simulink model "VCU_SW"  (R2020b)
settings: Solver=FixedStepDiscrete  StartTime=0.0  StopTime=inf  FixedStep=1e-2  RelTol=1e-3
PreLoadFcn:
  | RTWConfigurationCB('preloadfcn', bdroot);
InitFcn:
  | loadvar_ttc500
undefined symbols (not defined in the file): BrkPedalTypes, CabMovModeTypes, cFuseTempSensAcc_X, cFuseTempSensAcc_Y, cFuseTempSensVal_X, cFuseTempSensVal_Y, cTMSTempSensVal_X, cTMSTempSensVal_Y, cTransferCaseSpeedRatio, diag_state, DoorsPositionTypes, dP_filter_Y, DriverOccClassSystemTypes, ErrorValueTypes, fatal_error_callback, IO_ADC_NO_RANGE, LadderStatusTypes, pAnalogCabRotSensAcc, pAnalogCabRotSensMaxVolt, pAnalogCabRotSensMinVolt, pAnalogCabRotSensRange, pAnalogCabRotSensZeroVolt, pBrkActivePress, pCabTiltSensAcc, pCabTiltSensMaxCur, pCabTiltSensMinCur, pDistanceCorrection, pECANManual_BPNEnable, pECANManual_BPNEnabler_Flag, pFilterSensAccRes, pHDirMaxDiffFrq, pHDirSensHighLvl, pHDirSensLowLvl, pMainGearRatio, pMaxFilterSensRes, pMaxFirstPedalSensValue, pMaxFuseTempSensRes, pMaxPressLoss, pMaxPressSensCurrent, pMaxPressValue, pMaxPressValueHydMotAndPump, pMaxPressValueParkDrain, pMaxSecondPedalSensValue, pMaxTempSensVoltage, pMaxTempValue, pMaxTMSTempSensRes, pMinFilterSensRes, pMinFirstPedalSensValue, pMinFuseTempSensRes, pMinPressLoss, pMinPressSensCurrent, pMinPressValue, pMinSecondPedalSensValue, pMinTempSensVoltage, pMinTempValue, pMinTMSTempSensRes, pMotorRingTeethNum, pPedalSensAccuracyPct, pPedalSensAccuracyVolt, pPressLossTreshhold ... (+20)
libraries: TTlibrary x270, canmsglib x127, simulink x88
(part 11 of 17)

== system VCU_SW/InputLayer/InputNetwork/InputCCAN/GetCCAN100msec/CM3 ==
  CAN_Unpack_Cab_CM3 : canmsglib/CAN Unpack  MsgList=(none)  MsgName=CM3  MsgIDType=Extended (29-bit identifier)  MsgIdentifier=419288069  MsgLength=8  SignalInfo={ 'Transfer_Case_Selector_Switch', '0', '3', 'LE', 'unsigned', 'Standard', '0', '1', '0', '0', '7' }  IDPort=off  TimestampPort=off  ErrorPort=off  RemotePort=off  LengthPort=off  StatusPort=off  ApplyMinMax=off
      settings: SourceProductBaseCode=ME,XP,VN
  DataStoreWrite_PLC_StateM : DataStoreWrite  DataStoreName=InputNetworkData  DataStoreElements=InputNetworkData.CCAN.CM3.Transfer_Case_Selector_Switch
  MATLAB Function : MATLAB Function  TreatAsAtomicUnit=on
  Terminator : Terminator
  read_message_Cab_CM3 : TTlibrary/CAN/read_message_name  channel=IO_CAN_CHANNEL_1  id_format=IO_CAN_EXT_FRAME  get_msg_info=off  message_names=there is no CAN Unpack blocks  message_info=|  id=419288069  ac_mask=536870911  retranslation=off  io_error=on  sample_time=-1
      | Message Name: CM3
      |  Message ID Type: Extended (29-bit identifier)
      |  Message ID: 419288069
      settings: SourceProductName=TT control 500 series
  wires:
  MATLAB Function/1(TransferCaseEnum) -> DataStoreWrite_PLC_StateM/1
  CAN_Unpack_Cab_CM3/1 -> MATLAB Function/1(value)
  read_message_Cab_CM3/1 -> CAN_Unpack_Cab_CM3/1  "msg_419288069"
  read_message_Cab_CM3/2 -> Terminator/1  "handler_err_419288069"

== system VCU_SW/InputLayer/InputNetwork/InputCCAN/GetCCAN100msec/CabinAuxiliaryStatus ==
  CAN_Unpack_CabinAuxiliaryStatus : canmsglib/CAN Unpack  MsgList=(none)  MsgName=CabinAuxiliaryStatus  MsgIDType=Extended (29-bit identifier)  MsgIdentifier=419376638  MsgLength=8  SignalInfo={ 'FrameLockSts', '2', '2', 'LE', 'unsigned', 'Standard', '0', '1', '0', '0', '3'; 'FuelTankStatus', '0', '2', 'LE', 'unsigned', 'Standard', '0', '1', '0', '0', '3'; 'LadderStatus', '4', '2', 'LE', 'unsigned', 'Standard', '0', '1', '0', '0', '3' }  IDPort=off  TimestampPort=off  ErrorPort=off  RemotePort=off  LengthPort=off  StatusPort=off  ApplyMinMax=off
      settings: SourceProductBaseCode=ME,XP,VN
  DataStoreWrite_PLC_StateM : DataStoreWrite  DataStoreName=InputNetworkData  DataStoreElements=InputNetworkData.CCAN.CabinAuxiliaryStatus.FrameLockStatus#InputNetworkData.CCAN.CabinAuxiliaryStatus.FuelTankStatus#InputNetworkData.CCAN.CabinAuxiliaryStatus.LadderStatus
  Enumerated Constant1 : simulink/Sources/Enumerated Constant  OutDataTypeStr=Enum: StateModeTypes  Value=StateModeTypes.STT_DISABLE  SampleTime=inf
  Enumerated Constant8 : simulink/Sources/Enumerated Constant  OutDataTypeStr=Enum: LadderStatusTypes  Value=LadderStatusTypes.LADDER_UP  SampleTime=inf
  Function Caller1 : FunctionCaller  FunctionPrototype=rawValue = convUintPinToenumStt(uintValue)  InputArgumentSpecifications=<Enter example>  OutputArgumentSpecifications=<Enter example>
  Function Caller3 : FunctionCaller  FunctionPrototype=rawValue = convUintPinToenumStt(uintValue)  InputArgumentSpecifications=<Enter example>  OutputArgumentSpecifications=<Enter example>
  MATLAB Function : MATLAB Function  TreatAsAtomicUnit=on
  Terminator : Terminator
  read_message_CabinAuxiliaryStatus : TTlibrary/CAN/read_message_name  channel=IO_CAN_CHANNEL_1  id_format=IO_CAN_EXT_FRAME  get_msg_info=off  message_names=there is no CAN Unpack blocks  message_info=|  id=419376638  ac_mask=536870911  retranslation=off  io_error=on  sample_time=-1
      | Message Name: InstrumentClusterStatus
      |  Message ID Type: Extended (29-bit identifier)
      |  Message ID: 419384087
      settings: SourceProductName=TT control 500 series
  wires:
  read_message_CabinAuxiliaryStatus/2 -> Terminator/1  "handler_err_419376638"
  read_message_CabinAuxiliaryStatus/1 -> CAN_Unpack_CabinAuxiliaryStatus/1  "msg_419376638"
  CAN_Unpack_CabinAuxiliaryStatus/1 -> Function Caller3/1
  CAN_Unpack_CabinAuxiliaryStatus/3 -> MATLAB Function/1(Value)
  CAN_Unpack_CabinAuxiliaryStatus/2 -> Function Caller1/1
  Enumerated Constant1/1 -> DataStoreWrite_PLC_StateM/1
  Function Caller1/1 -> DataStoreWrite_PLC_StateM/2
  Enumerated Constant8/1 -> DataStoreWrite_PLC_StateM/3

== system VCU_SW/InputLayer/InputNetwork/InputCCAN/GetCCAN100msec/DC1 ==
  CAN_Unpack_Cab_DC1 : canmsglib/CAN Unpack  MsgList=(none)  MsgName=DC1  MsgIDType=Extended (29-bit identifier)  MsgIdentifier=419319550  MsgLength=8  SignalInfo={ 'PositionOfDoors', '0', '4', 'LE', 'unsigned', 'Standard', '0', '1', '0', '0', '15' }  IDPort=off  TimestampPort=off  ErrorPort=off  RemotePort=off  LengthPort=off  StatusPort=off  ApplyMinMax=off
      settings: SourceProductBaseCode=ME,XP,VN
  Data Store Write : DataStoreWrite  DataStoreName=InputFunctionsData  DataStoreElements=InputFunctionsData.doorIsClosed
  DataStoreWrite_PLC_StateM : DataStoreWrite  DataStoreName=InputNetworkData  DataStoreElements=InputNetworkData.CCAN.DC1.PositionOfDoors
  Enumerated Constant : simulink/Sources/Enumerated Constant  OutDataTypeStr=Enum: DoorsPositionTypes  Value=DoorsPositionTypes.DOORS_POS_ALL_DOORS_CLOSED  SampleTime=inf
  Enumerated Constant1 : simulink/Sources/Enumerated Constant  OutDataTypeStr=Enum: DoorsPositionTypes  Value=DoorsPositionTypes.DOORS_POS_ALL_DOORS_CLOSED  SampleTime=inf
  Enumerated Constant2 : simulink/Sources/Enumerated Constant  OutDataTypeStr=Enum: StateModeTypes  Value=StateModeTypes.STT_DISABLE  SampleTime=inf
  Enumerated Constant3 : simulink/Sources/Enumerated Constant  OutDataTypeStr=Enum: StateModeTypes  Value=StateModeTypes.STT_ENABLE  SampleTime=inf
  MATLAB Function : MATLAB Function  TreatAsAtomicUnit=on
  Multiport Switch : MultiPortSwitch  DataPortOrder=Zero-based contiguous  Inputs=2  zeroidx=on
  Relational Operator : RelationalOperator  Operator===  OutDataTypeStr=boolean  RndMeth=Simplest
  Terminator : Terminator
  read_message_Cab_DC1 : TTlibrary/CAN/read_message_name  channel=IO_CAN_CHANNEL_1  id_format=IO_CAN_EXT_FRAME  get_msg_info=off  message_names=there is no CAN Unpack blocks  message_info=|  id=419319550  ac_mask=536870911  retranslation=off  io_error=on  sample_time=-1
      | Message Name: DC1
      |  Message ID Type: Extended (29-bit identifier)
      |  Message ID: 419319550
      settings: SourceProductName=TT control 500 series
  wires:
  CAN_Unpack_Cab_DC1/1 -> MATLAB Function/1(Value)
  read_message_Cab_DC1/1 -> CAN_Unpack_Cab_DC1/1  "msg_419319550"
  read_message_Cab_DC1/2 -> Terminator/1  "handler_err_419319550"
  Enumerated Constant2/1 -> Multiport Switch/2
  Multiport Switch/1 -> Data Store Write/1  "closedDoorSensState"
  Relational Operator/1 -> Multiport Switch/1
  Enumerated Constant/1 -> DataStoreWrite_PLC_StateM/1, Relational Operator/1
  Enumerated Constant1/1 -> Relational Operator/2
  Enumerated Constant3/1 -> Multiport Switch/3  "closedDoorSensState"

== system VCU_SW/InputLayer/InputNetwork/InputCCAN/GetCCAN100msec/Fan Rotation Direction Control  ==
  CAN_Unpack_Cab_FanRotationDirectionControl : canmsglib/CAN Unpack  MsgList=(none)  MsgName=FanRotationDirectionControl  MsgIDType=Extended (29-bit identifier)  MsgIdentifier=419375365  MsgLength=8  SignalInfo={ 'FanDirectCmd', '0', '2', 'LE', 'unsigned', 'Standard', '0', '1', '0', '0', '3'; 'FanReverseCmd', '2', '2', 'LE', 'unsigned', 'Standard', '0', '1', '0', '0', '3' }  IDPort=off  TimestampPort=off  ErrorPort=off  RemotePort=off  LengthPort=off  StatusPort=off  ApplyMinMax=off
      settings: SourceProductBaseCode=ME,XP,VN
  DataStoreWrite_PLC_StateM : DataStoreWrite  DataStoreName=InputNetworkData  DataStoreElements=InputNetworkData.CCAN.FanRotationDirectionControl.FanDirectCmd#InputNetworkData.CCAN.FanRotationDirectionControl.FanReverseCmd
  Function Caller1 : FunctionCaller  FunctionPrototype=rawValue = convUintPinToenumStt(uintValue)  InputArgumentSpecifications=<Enter example>  OutputArgumentSpecifications=<Enter example>
  Function Caller2 : FunctionCaller  FunctionPrototype=rawValue = convUintPinToenumStt(uintValue)  InputArgumentSpecifications=<Enter example>  OutputArgumentSpecifications=<Enter example>
  Terminator : Terminator
  read_message_Cab_FanRotationDirectionControl : TTlibrary/CAN/read_message_name  channel=IO_CAN_CHANNEL_1  id_format=IO_CAN_EXT_FRAME  get_msg_info=off  message_names=there is no CAN Unpack blocks  message_info=|  id=419375365  ac_mask=536870911  retranslation=off  io_error=on  sample_time=-1
      | Message Name: FanRotationDirectionControl
      |  Message ID Type: Extended (29-bit identifier)
      |  Message ID: 419375365
      settings: SourceProductName=TT control 500 series
  wires:
  Function Caller2/1 -> DataStoreWrite_PLC_StateM/2
  Function Caller1/1 -> DataStoreWrite_PLC_StateM/1
  CAN_Unpack_Cab_FanRotationDirectionControl/2 -> Function Caller2/1
  CAN_Unpack_Cab_FanRotationDirectionControl/1 -> Function Caller1/1
  read_message_Cab_FanRotationDirectionControl/1 -> CAN_Unpack_Cab_FanRotationDirectionControl/1  "msg_419375365"
  read_message_Cab_FanRotationDirectionControl/2 -> Terminator/1  "handler_err_419375365"

== system VCU_SW/InputLayer/InputNetwork/InputCCAN/GetCCAN100msec/Fan Rotation Direction Status  ==
  CAN_Unpack_Cab_FanRotationDirectionStatus : canmsglib/CAN Unpack  MsgList=(none)  MsgName=FanRotationDirectionStatus  MsgIDType=Extended (29-bit identifier)  MsgIdentifier=419377150  MsgLength=8  SignalInfo={ 'FanDirectSts', '0', '2', 'LE', 'unsigned', 'Standard', '0', '1', '0', '0', '3'; 'FanReverseSts', '2', '2', 'LE', 'unsigned', 'Standard', '0', '1', '0', '0', '3' }  IDPort=off  TimestampPort=off  ErrorPort=off  RemotePort=off  LengthPort=off  StatusPort=off  ApplyMinMax=off
      settings: SourceProductBaseCode=ME,XP,VN
  DataStoreWrite_PLC_StateM : DataStoreWrite  DataStoreName=InputNetworkData  DataStoreElements=InputNetworkData.CCAN.FanRotationDirectionStatus.FanDirectSts#InputNetworkData.CCAN.FanRotationDirectionStatus.FanReverseSts
  Function Caller1 : FunctionCaller  FunctionPrototype=rawValue = convUintPinToenumStt(uintValue)  InputArgumentSpecifications=<Enter example>  OutputArgumentSpecifications=<Enter example>
  Function Caller2 : FunctionCaller  FunctionPrototype=rawValue = convUintPinToenumStt(uintValue)  InputArgumentSpecifications=<Enter example>  OutputArgumentSpecifications=<Enter example>
  Terminator : Terminator
  read_message_Cab_FanRotationDirectionStatus : TTlibrary/CAN/read_message_name  channel=IO_CAN_CHANNEL_1  id_format=IO_CAN_EXT_FRAME  get_msg_info=off  message_names=there is no CAN Unpack blocks  message_info=|  id=419377150  ac_mask=536870911  retranslation=off  io_error=on  sample_time=-1
      | Message Name: FanRotationDirectionStatus
      |  Message ID Type: Extended (29-bit identifier)
      |  Message ID: 419377150
      settings: SourceProductName=TT control 500 series
  wires:
  Function Caller1/1 -> DataStoreWrite_PLC_StateM/2
  Function Caller2/1 -> DataStoreWrite_PLC_StateM/1
  CAN_Unpack_Cab_FanRotationDirectionStatus/2 -> Function Caller1/1
  CAN_Unpack_Cab_FanRotationDirectionStatus/1 -> Function Caller2/1
  read_message_Cab_FanRotationDirectionStatus/1 -> CAN_Unpack_Cab_FanRotationDirectionStatus/1  "msg_419377150"
  read_message_Cab_FanRotationDirectionStatus/2 -> Terminator/1  "handler_err_419377150"

== system VCU_SW/InputLayer/InputNetwork/InputCCAN/GetCCAN100msec/FuelTankAndFrameLock ==
  CAN_Unpack_Cab_FuelTankAndFrameLock : canmsglib/CAN Unpack  MsgList=(none)  MsgName=FuelTankAndFrameLock  MsgIDType=Extended (29-bit identifier)  MsgIdentifier=419375621  MsgLength=8  SignalInfo={ 'FrameLockCmd', '2', '2', 'LE', 'unsigned', 'Standard', '0', '1', '0', '-Inf', 'Inf'; 'FuelTankSwitch', '0', '2', 'LE', 'unsigned', 'Standard', '0', '1', '0', '0', '3' }  IDPort=off  TimestampPort=off  ErrorPort=off  RemotePort=off  LengthPort=off  StatusPort=off  ApplyMinMax=off
      settings: SourceProductBaseCode=ME,XP,VN
  Data Store Write : DataStoreWrite  DataStoreName=InputNetworkData  DataStoreElements=InputNetworkData.CCAN.FuelTankAndFrameLock.FrameLockCmd#InputNetworkData.CCAN.FuelTankAndFrameLock.FuelTankSwitch
  Terminator : Terminator
  read_message_Cab_FuelTankAndFrameLock : TTlibrary/CAN/read_message_name  channel=IO_CAN_CHANNEL_1  id_format=IO_CAN_EXT_FRAME  get_msg_info=off  message_names=there is no CAN Unpack blocks  message_info=|  id=419375621  ac_mask=536870911  retranslation=off  io_error=on  sample_time=-1
      | Message Name: OWWStatus
      |  Message ID Type: Extended (29-bit identifier)
      |  Message ID: 419376894
      settings: SourceProductName=TT control 500 series
  wires:
  read_message_Cab_FuelTankAndFrameLock/2 -> Terminator/1  "handler_err_419375621"
  read_message_Cab_FuelTankAndFrameLock/1 -> CAN_Unpack_Cab_FuelTankAndFrameLock/1  "msg_419375621"
  CAN_Unpack_Cab_FuelTankAndFrameLock/2 -> Data Store Write/2
  CAN_Unpack_Cab_FuelTankAndFrameLock/1 -> Data Store Write/1

== system VCU_SW/InputLayer/InputNetwork/InputCCAN/GetCCAN100msec/Instrument Cluster Status  ==
  CAN_Unpack_Cab_InstrumentClusterStatus : canmsglib/CAN Unpack  MsgList=(none)  MsgName=InstrumentClusterStatus  MsgIDType=Extended (29-bit identifier)  MsgIdentifier=419384087  MsgLength=8  SignalInfo={ 'RearCameraEnaSts', '0', '2', 'LE', 'unsigned', 'Standard', '0', '1', '0', '0', '3' }  IDPort=off  TimestampPort=off  ErrorPort=off  RemotePort=off  LengthPort=off  StatusPort=off  ApplyMinMax=off
      settings: SourceProductBaseCode=ME,XP,VN
  DataStoreWrite_PLC_StateM : DataStoreWrite  DataStoreName=InputNetworkData  DataStoreElements=InputNetworkData.CCAN.InstrumentClusterStatus.RearCameraEnaSts
  Function Caller3 : FunctionCaller  FunctionPrototype=rawValue = convUintPinToenumStt(uintValue)  InputArgumentSpecifications=<Enter example>  OutputArgumentSpecifications=<Enter example>
  Terminator : Terminator
  read_message_Cab_InstrumentClusterStatus : TTlibrary/CAN/read_message_name  channel=IO_CAN_CHANNEL_1  id_format=IO_CAN_EXT_FRAME  get_msg_info=off  message_names=there is no CAN Unpack blocks  message_info=|  id=419384087  ac_mask=536870911  retranslation=off  io_error=on  sample_time=-1
      | Message Name: InstrumentClusterStatus
      |  Message ID Type: Extended (29-bit identifier)
      |  Message ID: 419384087
      settings: SourceProductName=TT control 500 series
  wires:
  CAN_Unpack_Cab_InstrumentClusterStatus/1 -> Function Caller3/1
  read_message_Cab_InstrumentClusterStatus/1 -> CAN_Unpack_Cab_InstrumentClusterStatus/1  "msg_419384087"
  read_message_Cab_InstrumentClusterStatus/2 -> Terminator/1  "handler_err_419384087"
  Function Caller3/1 -> DataStoreWrite_PLC_StateM/1

== system VCU_SW/InputLayer/InputNetwork/InputCCAN/GetCCAN100msec/Left Big Pan Cmd ==
  CAN_Unpack_Cab_LeftBigPanCmd : canmsglib/CAN Unpack  MsgList=(none)  MsgName=LeftBigPanCmd  MsgIDType=Extended (29-bit identifier)  MsgIdentifier=419380229  MsgLength=8  SignalInfo={ 'DecreaseCmd', '8', '2', 'LE', 'unsigned', 'Standard', '0', '1', '0', '0', '3'; 'DownCmd', '10', '2', 'LE', 'unsigned', 'Standard', '0', '1', '0', '0', '3'; 'EscapeCmd', '16', '2', 'LE', 'unsigned', 'Standard', '0', '1', '0', '0', '3'; 'IncreaseCmd', '6', '2', 'LE', 'unsigned', 'Standard', '0', '1', '0', '0', '3'; 'LeftCmd', '2', '2', 'LE', 'unsigned', 'Standard', '0', '1', '0', '0', '3'; 'OKCmd', '4', '2', 'LE', 'unsigned', 'Standard', '0', '1', '0', '0', '3'; 'ReturnCmd', '14', '2', 'LE', 'unsigned', 'Standard', '0', '1', '0', '0', '3'; 'RightCmd', '12', '2', 'LE', 'unsigned', 'Standard', '0', '1', '0', '0', '3'; 'UpCmd', '0', '2', 'LE', 'unsigned', 'Standard', '0', '1', '0', '0', '3' }  IDPort=off  TimestampPort=off  ErrorPort=off  RemotePort=off  LengthPort=off  StatusPort=off  ApplyMinMax=off
      settings: SourceProductBaseCode=ME,XP,VN
  DataStoreWrite_PLC_StateM : DataStoreWrite  DataStoreName=InputNetworkData  DataStoreElements=InputNetworkData.CCAN.LeftBigPanCmd.DecreaseCmd#InputNetworkData.CCAN.LeftBigPanCmd.DownCmd#InputNetworkData.CCAN.LeftBigPanCmd.EscapeCmd#InputNetworkData.CCAN.LeftBigPanCmd.IncreaseCmd#InputNetworkData.CCAN.LeftBigPanCmd.LeftCmd#InputNetworkData.CCAN.LeftBigPanCmd.OKCmd#InputNetworkData.CCAN.LeftBigPanCmd.ReturnCmd#InputNetworkData.CCAN.LeftBigPanCmd.RightCmd#InputNetworkData.CCAN.LeftBigPanCmd.UpCmd
  Function Caller{1..9} (9 alike) : FunctionCaller  FunctionPrototype=rawValue = convUintPinToenumStt(uintValue)  InputArgumentSpecifications=<Enter example>  OutputArgumentSpecifications=<Enter example>
  Terminator : Terminator
  read_message_Cab_LeftBigPanCmd : TTlibrary/CAN/read_message_name  channel=IO_CAN_CHANNEL_1  id_format=IO_CAN_EXT_FRAME  get_msg_info=off  message_names=there is no CAN Unpack blocks  message_info=|  id=419380229  ac_mask=536870911  retranslation=off  io_error=on  sample_time=-1
      | Message Name: NumKeyboardCmd
      |  Message ID Type: Extended (29-bit identifier)
      |  Message ID: 419380229
      settings: SourceProductName=TT control 500 series
  wires:
  read_message_Cab_LeftBigPanCmd/1 -> CAN_Unpack_Cab_LeftBigPanCmd/1  "msg_419380229"
  read_message_Cab_LeftBigPanCmd/2 -> Terminator/1  "handler_err_419380229"
  CAN_Unpack_Cab_LeftBigPanCmd/1 -> Function Caller1/1
  Function Caller1/1 -> DataStoreWrite_PLC_StateM/1
  Function Caller2/1 -> DataStoreWrite_PLC_StateM/2
  Function Caller3/1 -> DataStoreWrite_PLC_StateM/3
  Function Caller4/1 -> DataStoreWrite_PLC_StateM/4
  CAN_Unpack_Cab_LeftBigPanCmd/2 -> Function Caller2/1
  CAN_Unpack_Cab_LeftBigPanCmd/3 -> Function Caller3/1
  CAN_Unpack_Cab_LeftBigPanCmd/4 -> Function Caller4/1
  CAN_Unpack_Cab_LeftBigPanCmd/5 -> Function Caller5/1
  Function Caller5/1 -> DataStoreWrite_PLC_StateM/5
  Function Caller6/1 -> DataStoreWrite_PLC_StateM/6
  CAN_Unpack_Cab_LeftBigPanCmd/6 -> Function Caller6/1
  Function Caller7/1 -> DataStoreWrite_PLC_StateM/7
  CAN_Unpack_Cab_LeftBigPanCmd/7 -> Function Caller7/1
  Function Caller8/1 -> DataStoreWrite_PLC_StateM/8
  CAN_Unpack_Cab_LeftBigPanCmd/8 -> Function Caller8/1
  CAN_Unpack_Cab_LeftBigPanCmd/9 -> Function Caller9/1
  Function Caller9/1 -> DataStoreWrite_PLC_StateM/9

== system VCU_SW/InputLayer/InputNetwork/InputCCAN/GetCCAN100msec/Left Small Pan Cmd ==
  CAN_Unpack_Cab_LeftSmallPanCmd : canmsglib/CAN Unpack  MsgList=(none)  MsgName=LeftSmallPanCmd  MsgIDType=Extended (29-bit identifier)  MsgIdentifier=419377669  MsgLength=8  SignalInfo={ 'BoughCutting', '32', '2', 'LE', 'unsigned', 'Standard', '0', '1', '0', '0', '3'; 'EnableSaw', '30', '2', 'LE', 'unsigned', 'Standard', '0', '1', '0', '0', '3'; 'Num0BttnCmd', '18', '2', 'LE', 'unsigned', 'Standard', '0', '1', '0', '0', '3'; 'Num1BttnCmd', '0', '2', 'LE', 'unsigned', 'Standard', '0', '1', '0', '0', '3'; 'Num2BttnCmd', '2', '2', 'LE', 'unsigned', 'Standard', '0', '1', '0', '0', '3'; 'Num3BttnCmd', '4', '2', 'LE', 'unsigned', 'Standard', '0', '1', '0', '0', '3'; 'Num4BttnCmd', '6', '2', 'LE', 'unsigned', 'Standard', '0', '1', '0', '0', '3'; 'Num5BttnCmd', '8', '2', 'LE', 'unsigned', 'Standard', '0', '1', '0', '0', '3'; 'Num6BttnCmd', '10', '2', 'LE', 'unsigned', 'Standard', '0', '1', '0', '0', '3'; 'Num7BttnCmd', '12', '2', 'LE', 'unsigned', 'Standard', '0', '1', '0', '0', '3'; 'Num8BttnCmd', '14', '2', 'LE', 'unsigned', 'Standard', '0', '1', '0', '0', '3'; 'Num9BttnCmd', '16', '2', 'LE', 'unsigned', 'Standard', '0', '1', '0', '0', '3'; 'SelectAspenWood', '26', '2', 'LE', 'unsigned', 'Standard', '0', '1', '0', '0', '3'; 'SelectBirchWood', '24', '2', 'LE', 'unsigned', 'Standard', '0', '1', '0', '0', '3'; 'SelectNewTrunk', '28', '2', 'LE', 'unsigned', 'Standard', '0', '1', '0', '0', '3'; 'SelectPineWood', '22', '2', 'LE', 'unsigned', 'Standard', '0', '1', '0', '0', '3'; 'SelectSpruceWood', '20', '2', 'LE', 'unsigned', 'Standard', '0', '1', '0', '0', '3'; 'StumpProcessing', '34', '2', 'LE', 'unsigned', 'Standard', '0', '1', '0', '0', '3' }  IDPort=off  TimestampPort=off  ErrorPort=off  RemotePort=off  LengthPort=off  StatusPort=off  ApplyMinMax=off
      settings: SourceProductBaseCode=ME,XP,VN
  DataStoreWrite_PLC_StateM : DataStoreWrite  DataStoreName=InputNetworkData  DataStoreElements=InputNetworkData.CCAN.LeftSmallPanCmd.BoughCutting#InputNetworkData.CCAN.LeftSmallPanCmd.EnableSaw#InputNetworkData.CCAN.LeftSmallPanCmd.Num0BttnCmd#InputNetworkData.CCAN.LeftSmallPanCmd.Num1BttnCmd#InputNetworkData.CCAN.LeftSmallPanCmd.Num2BttnCmd#InputNetworkData.CCAN.LeftSmallPanCmd.Num3BttnCmd#InputNetworkData.CCAN.LeftSmallPanCmd.Num4BttnCmd#InputNetworkData.CCAN.LeftSmallPanCmd.Num5BttnCmd#InputNetworkData.CCAN.LeftSmallPanCmd.Num6BttnCmd#InputNetworkData.CCAN.LeftSmallPanCmd.Num7BttnCmd#InputNetworkData.CCAN.LeftSmallPanCmd.Num8BttnCmd#InputNetworkData.CCAN.LeftSmallPanCmd.Num9BttnCmd#InputNetworkData.CCAN.LeftSmallPanCmd.SelectAspenWood#InputNetworkData.CCAN.LeftSmallPanCmd.SelectBirchWood#InputNetworkData.CCAN.LeftSmallPanCmd.SelectNewTrunk#InputNetworkData.CCAN.LeftSmallPanCmd.SelectPineWood#InputNetworkData.CCAN.LeftSmallPanCmd.SelectSpruceWood#InputNetworkData.CCAN.LeftSmallPanCmd.StumpProcessing
  Function Caller{1..18} (18 alike) : FunctionCaller  FunctionPrototype=rawValue = convUintPinToenumStt(uintValue)  InputArgumentSpecifications=<Enter example>  OutputArgumentSpecifications=<Enter example>
  Terminator : Terminator
  read_message_Cab_LeftSmallPanCmd : TTlibrary/CAN/read_message_name  channel=IO_CAN_CHANNEL_1  id_format=IO_CAN_EXT_FRAME  get_msg_info=off  message_names=there is no CAN Unpack blocks  message_info=|  id=419377669  ac_mask=536870911  retranslation=off  io_error=on  sample_time=-1
      | Message Name: LumberProcessingCmd
      |  Message ID Type: Extended (29-bit identifier)
      |  Message ID: 419377669
      settings: SourceProductName=TT control 500 series
  wires:
  read_message_Cab_LeftSmallPanCmd/1 -> CAN_Unpack_Cab_LeftSmallPanCmd/1  "msg_419377669"
  read_message_Cab_LeftSmallPanCmd/2 -> Terminator/1  "handler_err_419377669"
  CAN_Unpack_Cab_LeftSmallPanCmd/1 -> Function Caller1/1
  Function Caller1/1 -> DataStoreWrite_PLC_StateM/1
  CAN_Unpack_Cab_LeftSmallPanCmd/2 -> Function Caller2/1
  Function Caller2/1 -> DataStoreWrite_PLC_StateM/2
  CAN_Unpack_Cab_LeftSmallPanCmd/3 -> Function Caller3/1
  Function Caller3/1 -> DataStoreWrite_PLC_StateM/3
  CAN_Unpack_Cab_LeftSmallPanCmd/4 -> Function Caller4/1
  Function Caller4/1 -> DataStoreWrite_PLC_StateM/4
  CAN_Unpack_Cab_LeftSmallPanCmd/5 -> Function Caller5/1
  Function Caller5/1 -> DataStoreWrite_PLC_StateM/5
  Function Caller6/1 -> DataStoreWrite_PLC_StateM/6
  CAN_Unpack_Cab_LeftSmallPanCmd/6 -> Function Caller6/1
  Function Caller7/1 -> DataStoreWrite_PLC_StateM/7
  CAN_Unpack_Cab_LeftSmallPanCmd/7 -> Function Caller7/1
  Function Caller8/1 -> DataStoreWrite_PLC_StateM/8
  CAN_Unpack_Cab_LeftSmallPanCmd/8 -> Function Caller8/1
  Function Caller9/1 -> DataStoreWrite_PLC_StateM/9
  CAN_Unpack_Cab_LeftSmallPanCmd/9 -> Function Caller9/1
  CAN_Unpack_Cab_LeftSmallPanCmd/10 -> Function Caller10/1
  Function Caller10/1 -> DataStoreWrite_PLC_StateM/10
  CAN_Unpack_Cab_LeftSmallPanCmd/11 -> Function Caller11/1
  Function Caller11/1 -> DataStoreWrite_PLC_StateM/11
  CAN_Unpack_Cab_LeftSmallPanCmd/12 -> Function Caller12/1
  Function Caller12/1 -> DataStoreWrite_PLC_StateM/12
  CAN_Unpack_Cab_LeftSmallPanCmd/13 -> Function Caller13/1
  Function Caller13/1 -> DataStoreWrite_PLC_StateM/13
  Function Caller14/1 -> DataStoreWrite_PLC_StateM/14
  CAN_Unpack_Cab_LeftSmallPanCmd/14 -> Function Caller14/1
  Function Caller15/1 -> DataStoreWrite_PLC_StateM/15
  CAN_Unpack_Cab_LeftSmallPanCmd/15 -> Function Caller15/1
  Function Caller16/1 -> DataStoreWrite_PLC_StateM/16
  CAN_Unpack_Cab_LeftSmallPanCmd/16 -> Function Caller16/1
  Function Caller17/1 -> DataStoreWrite_PLC_StateM/17
  CAN_Unpack_Cab_LeftSmallPanCmd/17 -> Function Caller17/1
  Function Caller18/1 -> DataStoreWrite_PLC_StateM/18
  CAN_Unpack_Cab_LeftSmallPanCmd/18 -> Function Caller18/1

== system VCU_SW/InputLayer/InputNetwork/InputCCAN/GetCCAN100msec/OWW Status  ==
  CAN_Unpack_Cab_OWWStatus : canmsglib/CAN Unpack  MsgList=(none)  MsgName=OWWStatus  MsgIDType=Extended (29-bit identifier)  MsgIdentifier=419376894  MsgLength=8  SignalInfo={ 'FrontOperatorWasherSts', '45', '3', 'LE', 'unsigned', 'Standard', '0', '1', '0', '0', '7'; 'FrontOperatorWiperSts', '4', '4', 'LE', 'unsigned', 'Standard', '0', '1', '0', '0', '15'; 'RearWasherFunctionSts', '53', '3', 'LE', 'unsigned', 'Standard', '0', '1', '0', '0', '7'; 'RearWiperSts', '12', '4', 'LE', 'unsigned', 'Standard', '0', '1', '0', '0', '15' }  IDPort=off  TimestampPort=off  ErrorPort=off  RemotePort=off  LengthPort=off  StatusPort=off  ApplyMinMax=off
      settings: SourceProductBaseCode=ME,XP,VN
  DataStoreWrite_PLC_StateM : DataStoreWrite  DataStoreName=InputNetworkData  DataStoreElements=InputNetworkData.CCAN.OWWStatus.FrontOperatorWasherSts#InputNetworkData.CCAN.OWWStatus.FrontOperatorWiperSts#InputNetworkData.CCAN.OWWStatus.RearWasherFunctionSts#InputNetworkData.CCAN.OWWStatus.RearWiperSts
  Terminator : Terminator
  read_message_Cab_OWWStatus : TTlibrary/CAN/read_message_name  channel=IO_CAN_CHANNEL_1  id_format=IO_CAN_EXT_FRAME  get_msg_info=off  message_names=there is no CAN Unpack blocks  message_info=|  id=419376894  ac_mask=536870911  retranslation=off  io_error=on  sample_time=-1
      | Message Name: OWWStatus
      |  Message ID Type: Extended (29-bit identifier)
      |  Message ID: 419376894
      settings: SourceProductName=TT control 500 series
  wires:
  CAN_Unpack_Cab_OWWStatus/4 -> DataStoreWrite_PLC_StateM/4
  CAN_Unpack_Cab_OWWStatus/3 -> DataStoreWrite_PLC_StateM/3
  CAN_Unpack_Cab_OWWStatus/2 -> DataStoreWrite_PLC_StateM/2
  CAN_Unpack_Cab_OWWStatus/1 -> DataStoreWrite_PLC_StateM/1
  read_message_Cab_OWWStatus/1 -> CAN_Unpack_Cab_OWWStatus/1  "msg_419376894"
  read_message_Cab_OWWStatus/2 -> Terminator/1  "handler_err_419376894"

== system VCU_SW/InputLayer/InputNetwork/InputCCAN/GetCCAN100msec/PTO ==
  CAN_Unpack_Cab_PTO : canmsglib/CAN Unpack  MsgList=(none)  MsgName=PTO  MsgIDType=Extended (29-bit identifier)  MsgIdentifier=419360773  MsgLength=8  SignalInfo={ 'EngPTO_GvrnrEnaSwtch', '40', '2', 'LE', 'unsigned', 'Standard', '0', '1', '0', '0', '3' }  IDPort=off  TimestampPort=off  ErrorPort=off  RemotePort=off  LengthPort=off  StatusPort=off  ApplyMinMax=off
      settings: SourceProductBaseCode=ME,XP,VN
  DataStoreWrite_PLC_StateM : DataStoreWrite  DataStoreName=InputNetworkData  DataStoreElements=InputNetworkData.CCAN.PTO.EngPTO_GvrnrEnaSwtch
  Function Caller1 : FunctionCaller  FunctionPrototype=rawValue = convUintPinToenumStt(uintValue)  InputArgumentSpecifications=<Enter example>  OutputArgumentSpecifications=<Enter example>
  Terminator : Terminator
  read_message_Cab_PTO : TTlibrary/CAN/read_message_name  channel=IO_CAN_CHANNEL_1  id_format=IO_CAN_EXT_FRAME  get_msg_info=off  message_names=there is no CAN Unpack blocks  message_info=|  id=419360773  ac_mask=536870911  retranslation=off  io_error=on  sample_time=-1
      | Message Name: PTO
      |  Message ID Type: Extended (29-bit identifier)
      |  Message ID: 419360773
      settings: SourceProductName=TT control 500 series
  wires:
  Function Caller1/1 -> DataStoreWrite_PLC_StateM/1
  CAN_Unpack_Cab_PTO/1 -> Function Caller1/1
  read_message_Cab_PTO/1 -> CAN_Unpack_Cab_PTO/1  "msg_419360773"
  read_message_Cab_PTO/2 -> Terminator/1  "handler_err_419360773"

== system VCU_SW/InputLayer/InputNetwork/InputCCAN/GetCCAN100msec/Remote Brake Command  ==
  CAN_Unpack_Cab_RemoteCommand : canmsglib/CAN Unpack  MsgList=(none)  MsgName=RemoteBrakeCommand  MsgIDType=Extended (29-bit identifier)  MsgIdentifier=218044421  MsgLength=8  SignalInfo={ 'RemoteBrakeButtonStatus', '0', '2', 'LE', 'unsigned', 'Standard', '0', '1', '0', '0', '3' }  IDPort=off  TimestampPort=off  ErrorPort=off  RemotePort=off  LengthPort=off  StatusPort=off  ApplyMinMax=off
      settings: SourceProductBaseCode=ME,XP,VN
  DataStoreWrite_PLC_StateM : DataStoreWrite  DataStoreName=InputNetworkData  DataStoreElements=InputNetworkData.CCAN.RemoteBrakeCommand.RemoteBrakeButtonStatus
  Function Caller1 : FunctionCaller  FunctionPrototype=rawValue = convUintPinToenumStt(uintValue)  InputArgumentSpecifications=<Enter example>  OutputArgumentSpecifications=<Enter example>
  Terminator : Terminator
  read_message_Cab_RemoteBrakeCommand : TTlibrary/CAN/read_message_name  channel=IO_CAN_CHANNEL_1  id_format=IO_CAN_EXT_FRAME  get_msg_info=off  message_names=there is no CAN Unpack blocks  message_info=|  id=218044421  ac_mask=536870911  retranslation=off  io_error=on  sample_time=-1
      | Message Name: RemoteBrakeCommand
      |  Message ID Type: Extended (29-bit identifier)
      |  Message ID: 218044421
      settings: SourceProductName=TT control 500 series
  wires:
  Function Caller1/1 -> DataStoreWrite_PLC_StateM/1
  CAN_Unpack_Cab_RemoteCommand/1 -> Function Caller1/1
  read_message_Cab_RemoteBrakeCommand/1 -> CAN_Unpack_Cab_RemoteCommand/1  "msg_218044421"
  read_message_Cab_RemoteBrakeCommand/2 -> Terminator/1  "handler_err_218044421"

== system VCU_SW/InputLayer/InputNetwork/InputCCAN/GetCCAN100msec/Right Small Pan Cmd ==
  CAN_Unpack_Cab_RightSmallPanCmd : canmsglib/CAN Unpack  MsgList=(none)  MsgName=RightSmallPanCmd  MsgIDType=Extended (29-bit identifier)  MsgIdentifier=419375109  MsgLength=8  SignalInfo={ 'HornSwitch', '2', '2', 'LE', 'unsigned', 'Standard', '0', '1', '0', '0', '3'; 'LadderSwitch', '4', '2', 'LE', 'unsigned', 'Standard', '0', '1', '0', '0', '3'; 'ManipTableLeanBackward', '8', '2', 'LE', 'unsigned', 'Standard', '0', '1', '0', '0', '3'; 'ManipTableLeanForward', '6', '2', 'LE', 'unsigned', 'Standard', '0', '1', '0', '0', '3'; 'ManipulatorEnable', '10', '2', 'LE', 'unsigned', 'Standard', '0', '1', '0', '0', '3'; 'RearCamEnaCmd', '0', '2', 'LE', 'unsigned', 'Standard', '0', '1', '0', '0', '3' }  IDPort=off  TimestampPort=off  ErrorPort=off  RemotePort=off  LengthPort=off  StatusPort=off  ApplyMinMax=off
      settings: SourceProductBaseCode=ME,XP,VN
  DataStoreWrite_PLC_StateM : DataStoreWrite  DataStoreName=InputNetworkData  DataStoreElements=InputNetworkData.CCAN.RightSmallPanCmd.HornSwitch#InputNetworkData.CCAN.RightSmallPanCmd.LadderSwitch#InputNetworkData.CCAN.RightSmallPanCmd.ManipTableLeanBackward#InputNetworkData.CCAN.RightSmallPanCmd.ManipTableLeanForward#InputNetworkData.CCAN.RightSmallPanCmd.ManipulatorEnable#InputNetworkData.CCAN.RightSmallPanCmd.RearCamEnaCmd
  Function Caller{1..5} (5 alike) : FunctionCaller  FunctionPrototype=rawValue = convUintPinToenumStt(uintValue)  InputArgumentSpecifications=<Enter example>  OutputArgumentSpecifications=<Enter example>
  MATLAB Function : MATLAB Function  TreatAsAtomicUnit=on
  Terminator : Terminator
  read_message_Cab_RightSmallPanCmd : TTlibrary/CAN/read_message_name  channel=IO_CAN_CHANNEL_1  id_format=IO_CAN_EXT_FRAME  get_msg_info=off  message_names=there is no CAN Unpack blocks  message_info=|  id=419375109  ac_mask=536870911  retranslation=off  io_error=on  sample_time=-1
      | Message Name: CabineAuxiliaryControl
      |  Message ID Type: Extended (29-bit identifier)
      |  Message ID: 419375109
      settings: SourceProductName=TT control 500 series
  wires:
  Function Caller3/1 -> DataStoreWrite_PLC_StateM/3
  CAN_Unpack_Cab_RightSmallPanCmd/3 -> Function Caller3/1
  Function Caller2/1 -> DataStoreWrite_PLC_StateM/4
  MATLAB Function/1(LadderStatus) -> DataStoreWrite_PLC_StateM/2
  CAN_Unpack_Cab_RightSmallPanCmd/5 -> Function Caller4/1
  CAN_Unpack_Cab_RightSmallPanCmd/4 -> Function Caller2/1
  CAN_Unpack_Cab_RightSmallPanCmd/2 -> MATLAB Function/1(Value)
  read_message_Cab_RightSmallPanCmd/1 -> CAN_Unpack_Cab_RightSmallPanCmd/1  "msg_419375109"
  read_message_Cab_RightSmallPanCmd/2 -> Terminator/1  "handler_err_419375109"
  CAN_Unpack_Cab_RightSmallPanCmd/1 -> Function Caller1/1
  Function Caller1/1 -> DataStoreWrite_PLC_StateM/1
  Function Caller4/1 -> DataStoreWrite_PLC_StateM/5
  CAN_Unpack_Cab_RightSmallPanCmd/6 -> Function Caller5/1
  Function Caller5/1 -> DataStoreWrite_PLC_StateM/6

== system VCU_SW/InputLayer/InputNetwork/InputCCAN/GetCCAN100msec/TC1 ==
  CAN_Unpack_Cab_BJM2 : canmsglib/CAN Unpack  MsgList=(none)  MsgName=TC1  MsgIDType=Extended (29-bit identifier)  MsgIdentifier=201456133  MsgLength=8  SignalInfo={ 'Trans_Mode_1', '40', '2', 'LE', 'unsigned', 'Standard', '0', '1', '0', '0', '3'; 'Trans_Mode_2', '42', '2', 'LE', 'unsigned', 'Standard', '0', '1', '0', '0', '3'; 'Trans_Mode_3', '44', '2', 'LE', 'unsigned', 'Standard', '0', '1', '0', '0', '3'; 'Trans_Requested_Gear', '16', '8', 'LE', 'unsigned', 'Standard', '0', '1', '0', '0', '255' }  IDPort=off  TimestampPort=off  ErrorPort=off  RemotePort=off  LengthPort=off  StatusPort=off  ApplyMinMax=off
      settings: SourceProductBaseCode=ME,XP,VN
  DataStoreWrite_PLC_StateM : DataStoreWrite  DataStoreName=InputNetworkData  DataStoreElements=InputNetworkData.CCAN.TC1.Trans_Mode_1#InputNetworkData.CCAN.TC1.Trans_Mode_2#InputNetworkData.CCAN.TC1.Trans_Mode_3#InputNetworkData.CCAN.TC1.Trans_Requested_Gear
  Function Caller1 : FunctionCaller  FunctionPrototype=rawValue = convUintPinToenumStt(uintValue)  InputArgumentSpecifications=<Enter example>  OutputArgumentSpecifications=<Enter example>
  Function Caller2 : FunctionCaller  FunctionPrototype=rawValue = convUintPinToenumStt(uintValue)  InputArgumentSpecifications=<Enter example>  OutputArgumentSpecifications=<Enter example>
  Function Caller3 : FunctionCaller  FunctionPrototype=rawValue = convUintPinToenumStt(uintValue)  InputArgumentSpecifications=<Enter example>  OutputArgumentSpecifications=<Enter example>
  MATLAB Function : MATLAB Function  TreatAsAtomicUnit=on
  Terminator : Terminator
  read_message_Cab_BJM2 : TTlibrary/CAN/read_message_name  channel=IO_CAN_CHANNEL_1  id_format=IO_CAN_EXT_FRAME  get_msg_info=off  message_names=there is no CAN Unpack blocks  message_info=|  id=201456133  ac_mask=536870911  retranslation=off  io_error=on  sample_time=-1
      | Message Name: TC1
      |  Message ID Type: Extended (29-bit identifier)
      |  Message ID: 201456133
      settings: SourceProductName=TT control 500 series
  wires:
  Function Caller3/1 -> DataStoreWrite_PLC_StateM/3
  Function Caller2/1 -> DataStoreWrite_PLC_StateM/2
  Function Caller1/1 -> DataStoreWrite_PLC_StateM/1
  MATLAB Function/1(leverPosEnum) -> DataStoreWrite_PLC_StateM/4
  CAN_Unpack_Cab_BJM2/4 -> MATLAB Function/1(value)
  CAN_Unpack_Cab_BJM2/3 -> Function Caller3/1
  CAN_Unpack_Cab_BJM2/2 -> Function Caller2/1
  CAN_Unpack_Cab_BJM2/1 -> Function Caller1/1
  read_message_Cab_BJM2/1 -> CAN_Unpack_Cab_BJM2/1  "msg_201456133"
  read_message_Cab_BJM2/2 -> Terminator/1  "handler_err_201456133"

== system VCU_SW/InputLayer/InputNetwork/InputCCAN/GetCCAN200msec/OWW ==
  CAN_Unpack_PLC_StateM : canmsglib/CAN Unpack  MsgList=(none)  MsgName=OWW  MsgIDType=Extended (29-bit identifier)  MsgIdentifier=419286277  MsgLength=8  SignalInfo={ 'FrontOperatorWasherSwtch', '45', '3', 'LE', 'unsigned', 'Standard', '0', '1', '0', '0', '7'; 'FrontOperatorWiperSwtch', '4', '4', 'LE', 'unsigned', 'Standard', '0', '1', '0', '0', '15'; 'RearWasherFunction', '53', '3', 'LE', 'unsigned', 'Standard', '0', '1', '0', '0', '7'; 'RearWiperSwtch', '12', '4', 'LE', 'unsigned', 'Standard', '0', '1', '0', '0', '15' }  IDPort=off  TimestampPort=off  ErrorPort=off  RemotePort=off  LengthPort=off  StatusPort=off  ApplyMinMax=off
      settings: SourceProductBaseCode=ME,XP,VN
  DataStoreWrite_PLC_StateM : DataStoreWrite  DataStoreName=InputNetworkData  DataStoreElements=InputNetworkData.CCAN.OWW.FrontOperatorWasherSwtch#InputNetworkData.CCAN.OWW.FrontOperatorWiperSwtch#InputNetworkData.CCAN.OWW.RearWasherFunction#InputNetworkData.CCAN.OWW.RearWiperSwtch
  Terminator : Terminator
  read_message_PLC_StateM : TTlibrary/CAN/read_message_name  channel=IO_CAN_CHANNEL_1  id_format=IO_CAN_EXT_FRAME  get_msg_info=off  message_names=there is no CAN Unpack blocks  message_info=|  id=419286277  ac_mask=536870911  retranslation=off  io_error=on  sample_time=-1
      | Message Name: OWW
      |  Message ID Type: Extended (29-bit identifier)
      |  Message ID: 419286277
      settings: SourceProductName=TT control 500 series
  wires:
  CAN_Unpack_PLC_StateM/4 -> DataStoreWrite_PLC_StateM/4
  CAN_Unpack_PLC_StateM/3 -> DataStoreWrite_PLC_StateM/3
  CAN_Unpack_PLC_StateM/2 -> DataStoreWrite_PLC_StateM/2
  CAN_Unpack_PLC_StateM/1 -> DataStoreWrite_PLC_StateM/1
  read_message_PLC_StateM/2 -> Terminator/1  "handler_err_419286277"
  read_message_PLC_StateM/1 -> CAN_Unpack_PLC_StateM/1  "msg_419286277"

== system VCU_SW/InputLayer/InputNetwork/InputCCAN/GetCCAN500msec/EAC1 ==
  CAN_Unpack_PLC_StateM : canmsglib/CAN Unpack  MsgList=(none)  MsgName=EAC1  MsgIDType=Extended (29-bit identifier)  MsgIdentifier=418383365  MsgLength=8  SignalInfo={ 'Diff_LockState_CenReal', '28', '2', 'LE', 'unsigned', 'Standard', '0', '1', '0', '0', '3'; 'Differential_LockState_CenFront', '26', '2', 'LE', 'unsigned', 'Standard', '0', '1', '0', '0', '3'; 'Differential_LockState_Central', '24', '2', 'LE', 'unsigned', 'Standard', '0', '1', '0', '0', '3' }  IDPort=off  TimestampPort=off  ErrorPort=off  RemotePort=off  LengthPort=off  StatusPort=off  ApplyMinMax=off
      settings: SourceProductBaseCode=ME,XP,VN
  DataStoreWrite_PLC_StateM : DataStoreWrite  DataStoreName=InputNetworkData  DataStoreElements=InputNetworkData.CCAN.EAC1_in.Diff_LockState_CenRear#InputNetworkData.CCAN.EAC1_in.Differential_LockState_CenFront#InputNetworkData.CCAN.EAC1_in.Differential_LockState_Central
  Function Caller1 : FunctionCaller  FunctionPrototype=rawValue = convUintPinToenumStt(uintValue)  InputArgumentSpecifications=<Enter example>  OutputArgumentSpecifications=<Enter example>
  Function Caller2 : FunctionCaller  FunctionPrototype=rawValue = convUintPinToenumStt(uintValue)  InputArgumentSpecifications=<Enter example>  OutputArgumentSpecifications=<Enter example>
  Function Caller3 : FunctionCaller  FunctionPrototype=rawValue = convUintPinToenumStt(uintValue)  InputArgumentSpecifications=<Enter example>  OutputArgumentSpecifications=<Enter example>
  Terminator : Terminator
  read_message_PLC_StateM : TTlibrary/CAN/read_message_name  channel=IO_CAN_CHANNEL_1  id_format=IO_CAN_EXT_FRAME  get_msg_info=off  message_names=there is no CAN Unpack blocks  message_info=|  id=418383365  ac_mask=536870911  retranslation=off  io_error=on  sample_time=-1
      | Message Name: EAC1
      |  Message ID Type: Extended (29-bit identifier)
      |  Message ID: 418383365
      settings: SourceProductName=TT control 500 series
  wires:
  Function Caller3/1 -> DataStoreWrite_PLC_StateM/3
  Function Caller2/1 -> DataStoreWrite_PLC_StateM/2
  Function Caller1/1 -> DataStoreWrite_PLC_StateM/1
  CAN_Unpack_PLC_StateM/3 -> Function Caller3/1
  CAN_Unpack_PLC_StateM/2 -> Function Caller2/1
  CAN_Unpack_PLC_StateM/1 -> Function Caller1/1
  read_message_PLC_StateM/2 -> Terminator/1  "handler_err_418383365"
  read_message_PLC_StateM/1 -> CAN_Unpack_PLC_StateM/1  "msg_418383365"

== system VCU_SW/InputLayer/InputNetwork/InputDiagCAN/GetDiagCAN10msec/Simulink Function ==
  note: v oid V CU_SW_getUDSMsgSts ( u byte2 * r ty_serviceSts )
      | {
      | / * local block i/o variables */
      | u byte2 r tb_read_message_uds_handler_rx ;
      | / * S-Function (canMsgStatusGet_ttc500): ' < S349>/getMessageObjectStatus ' */
      | / / Get message object read_message_UDS_handler_rx status
      | r tb_read_message_uds_handler_rx = I O_CAN_MsgStatus ( r ead_message_UDS_handler_rx ) ; / * SignalConversion generated from: ' < S349>/y ' */
      | * r ty_serviceSts = r tb_read_message_uds_handler_rx ;
      | }
  getUDSMsgSts : TriggerPort  TriggerType=function-call  IsSimulinkFunction=on  FunctionName=getUDSMsgSts  FunctionVisibility=scoped  VariantControl=(inherit)
  getMessageObjectStatus : TTlibrary/CAN/getMessageObjectStatus  handler=transmit_message_vlvcmd_hyd1_handler_tx  sample_time=-1
      settings: SourceProductName=TT control 500 series
  y : ArgOut  DisableCoverage=on  OutDataTypeStr=uint16  ArgumentName=serviceSts
  wires:
  getMessageObjectStatus/1 -> y/1  "transmit_message_dd_vcu_handler_tx_status"

== system VCU_SW/InputLayer/InputNetwork/InputDiagCAN/GetDiagCAN10msec/Simulink Function1 ==
  parsingUDSMsg : TriggerPort  TriggerType=function-call  IsSimulinkFunction=on  FunctionName=parsingUDSMsg  FunctionVisibility=scoped  VariantControl=(inherit)
  CAN_Unpack_UDS : canmsglib/CAN Unpack  MsgList=(none)  MsgName=UDS  MsgIDType=Extended (29-bit identifier)  MsgIdentifier=215677463  MsgLength=8  SignalInfo={ 'Sevice_id', '0', '8', 'LE', 'unsigned', 'Standard', '0', '1', '0', '0', '255'; 'DataIdentifier', '8', '16', 'LE', 'unsigned', 'Standard', '0', '1', '0', '0', '65535'; 'DataRecord', '24', '16', 'LE', 'unsigned', 'Standard', '0', '1', '0', '0', '65535' }  IDPort=off  TimestampPort=off  ErrorPort=off  RemotePort=off  LengthPort=off  StatusPort=off  ApplyMinMax=off
      settings: SourceProductBaseCode=ME,XP,VN
  Data Store Write : DataStoreWrite  DataStoreName=UDSStruct  DataStoreElements=UDSStruct.Service_id#UDSStruct.DataIdentifier#UDSStruct.DataRecord
  Terminator1 : Terminator
  read_message_UDS : TTlibrary/CAN/read_message_name  channel=IO_CAN_CHANNEL_1  id_format=IO_CAN_EXT_FRAME  get_msg_info=off  message_names=there is no CAN Unpack blocks  message_info=|  id=215677463  ac_mask=536870911  retranslation=off  io_error=on  sample_time=-1
      | Message Name: PLC_StateM
      |  Message ID Type: Extended (29-bit identifier)
      |  Message ID: 419388800
      settings: SourceProductName=TT control 500 series
  wires:
  read_message_UDS/2 -> Terminator1/1  "handler_err_215677463"
  read_message_UDS/1 -> CAN_Unpack_UDS/1  "msg_215677463"
  CAN_Unpack_UDS/1 -> Data Store Write/1
  CAN_Unpack_UDS/2 -> Data Store Write/2
  CAN_Unpack_UDS/3 -> Data Store Write/3

== system VCU_SW/InputLayer/InputNetwork/InputDiagCAN/GetDiagCAN10msec/Simulink Function2 ==
  getWriteMsg : TriggerPort  TriggerType=function-call  IsSimulinkFunction=on  FunctionName=getWriteMsg  FunctionVisibility=scoped  VariantControl=(inherit)
  MATLAB Function2 : MATLAB Function  TreatAsAtomicUnit=on

== system VCU_SW/InputLayer/InputNetwork/InputDiagCAN/GetDiagCAN10msec1/Simulink Function1 ==
  parsingUDSMsg : TriggerPort  TriggerType=function-call  IsSimulinkFunction=on  FunctionName=parsingUDSMsg  FunctionVisibility=scoped  VariantControl=(inherit)
  CAN_Unpack_UDS : canmsglib/CAN Unpack  MsgList=(none)  MsgName=UDS  MsgIDType=Extended (29-bit identifier)  MsgIdentifier=215677463  MsgLength=8  SignalInfo={ 'Sevice_id', '0', '8', 'LE', 'unsigned', 'Standard', '0', '1', '0', '0', '255'; 'DataIdentifier', '8', '16', 'LE', 'unsigned', 'Standard', '0', '1', '0', '0', '65535'; 'DataRecord', '24', '16', 'LE', 'unsigned', 'Standard', '0', '1', '0', '0', '65535' }  IDPort=off  TimestampPort=off  ErrorPort=off  RemotePort=off  LengthPort=off  StatusPort=off  ApplyMinMax=off
      settings: SourceProductBaseCode=ME,XP,VN
  Data Store Read1 : DataStoreRead  DataStoreName=UDSStruct  DataStoreElements=UDSStruct.Service_id
  Data Store Read2 : DataStoreRead  DataStoreName=UDSStruct  DataStoreElements=UDSStruct.DataIdentifier
  Data Store Read3 : DataStoreRead  DataStoreName=UDSStruct  DataStoreElements=UDSStruct.DataRecord
  Data Store Write : DataStoreWrite  DataStoreName=UDSStruct  DataStoreElements=UDSStruct.Service_id#UDSStruct.DataIdentifier#UDSStruct.DataRecord
  Data Store Write2 : DataStoreWrite  DataStoreName=UDSStruct  DataStoreElements=UDSStruct.readUDSmsgFlag
  Data Type Conversion : DataTypeConversion  OutDataTypeStr=uint8
  Data Type Conversion1 : DataTypeConversion  OutDataTypeStr=uint16
  Data Type Conversion2 : DataTypeConversion  OutDataTypeStr=uint16
  MATLAB Function : MATLAB Function  TreatAsAtomicUnit=on
  Multiport Switch : MultiPortSwitch  DataPortOrder=Zero-based contiguous  Inputs=2  zeroidx=on
  Multiport Switch1 : MultiPortSwitch  DataPortOrder=Zero-based contiguous  Inputs=2  zeroidx=on
  Multiport Switch2 : MultiPortSwitch  DataPortOrder=Zero-based contiguous  Inputs=2  zeroidx=on
  read_message_UDS : TTlibrary/CAN/read_message_name  channel=IO_CAN_CHANNEL_1  id_format=IO_CAN_EXT_FRAME  get_msg_info=off  message_names=there is no CAN Unpack blocks  message_info=|  id=215677463  ac_mask=536870911  retranslation=off  io_error=on  sample_time=-1
      | Message Name: PLC_StateM
      |  Message ID Type: Extended (29-bit identifier)
      |  Message ID: 419388800
      settings: SourceProductName=TT control 500 series
  wires:
  CAN_Unpack_UDS/3 -> Data Type Conversion2/1
  Multiport Switch/1 -> Data Store Write/1
  read_message_UDS/1 -> CAN_Unpack_UDS/1  "msg_215677463"
  CAN_Unpack_UDS/2 -> Data Type Conversion1/1
  Data Store Read2/1 -> Multiport Switch1/3
  Data Store Read3/1 -> Multiport Switch2/3
  CAN_Unpack_UDS/1 -> Data Type Conversion/1
  read_message_UDS/2 -> Multiport Switch2/1, Multiport Switch1/1, Multiport Switch/1, MATLAB Function/1(errSts)  "handler_err_215677463"
  Multiport Switch2/1 -> Data Store Write/3
  Multiport Switch1/1 -> Data Store Write/2
  Data Store Read1/1 -> Multiport Switch/3
  Data Type Conversion/1 -> Multiport Switch/2
  Data Type Conversion1/1 -> Multiport Switch1/2
  Data Type Conversion2/1 -> Multiport Switch2/2
  MATLAB Function/1(ReadUDSmsgFlag) -> Data Store Write2/1

== system VCU_SW/InputLayer/InputNetwork/InputDiagCAN/GetDiagCAN10msec1/Simulink Function2 ==
  getWriteMsg : TriggerPort  TriggerType=function-call  IsSimulinkFunction=on  FunctionName=getWriteMsg  FunctionVisibility=scoped  VariantControl=(inherit)
  MATLAB Function2 : MATLAB Function  TreatAsAtomicUnit=on
